simulink model "ElectroHydraulicActuator"  (R2024b)
settings: Solver=VariableStepAuto  StartTime=0.0  StopTime=25  RelTol=1e-3
undefined symbols (not defined in the file or in its folder): B, J, Ke, Kt, L, R
libraries: SignalEditorBlockLib x1
settings Model: Creator=eshwa  LastModifiedBy=eshwa

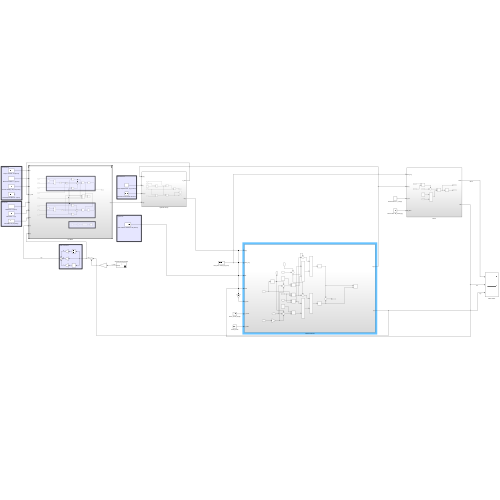
[thumbnail: Simulink's stored preview of the top-level diagram]
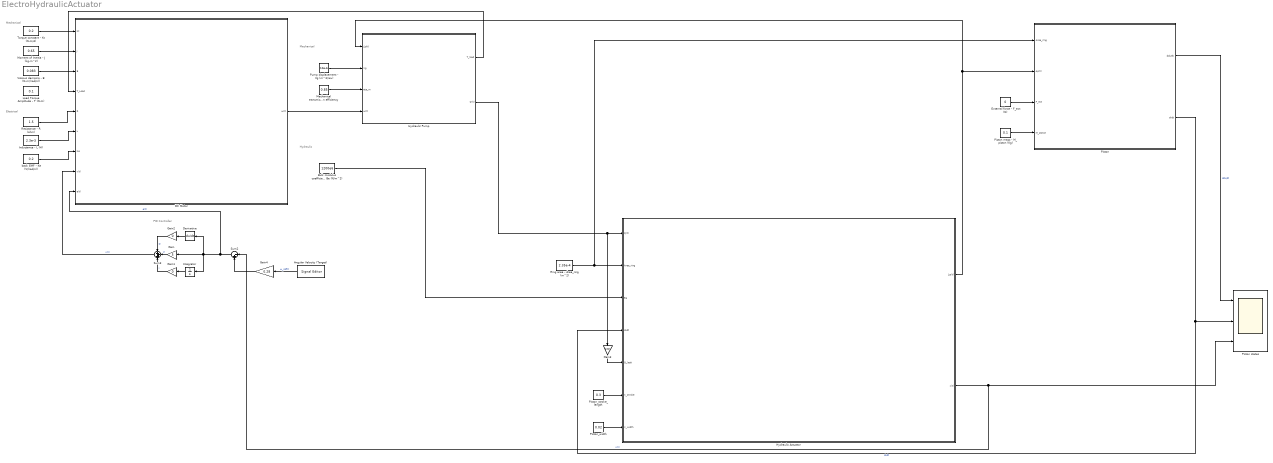
== system ElectroHydraulicActuator ==
  note: Mechanical
  note: PID Controller
  note: Mechanical
  note: Electrical
  note: Hydraulic
  Angular Velocity (Target) : SignalEditorBlockLib/Signal Editor  FileName=omega_ref.mat  ActiveScenario=Scenario  ActiveSignal=Ramp  IsBus=off  OutputBusObjectStr=Bus: BusObject  SampleTime=0  Interpolate=off  ZeroCross=off  OutputAfterFinalValue=Setting to zero  Unit=inherit  PreserveSignalName=on  ApplySigPropsToAllScenarios=on  ApplySigPropsToAllSignals=off
  Bulk modulus coefficient - Be (N/m^2) : Constant  Value=1200e6
  DC Motor : Subsystem
  Derivative : Derivative
  External force - F_ext (N) : Constant  Value=0
  Gain : Gain  Gain=5
  Gain1 : Gain  Gain=0
  Gain2 : Gain  Gain=0
  Gain3 : Gain  Gain=0.02
  Gain4 : Gain  Gain=0.28
  Hydraulic Actuator : Subsystem
  Hydraulic Pump : Subsystem
  Inductance - L (H) : Constant  Value=2.3e-3
  Integrator : Integrator
  Load Torque Amplitude - T (N-m) : Constant  Value=0.1
  Mechanical transmission efficiency : Constant  Value=0.85
  Moment of Inertia - J (kg-m^2) : Constant  Value=0.65
  Piston : Subsystem
  Piston mass - M_piston (Kg) : Constant  Value=0.1
  Piston states : Scope  NumInputPorts=3
  Piston_stroke_length : Constant  Value=0.3
  Piston_width : Constant  Value=0.02
  Pump displacement - Vg (m^3/rev) : Constant  Value=10e-6
  Resistance - R (ohm) : Constant  Value=1.5
  Ring area - Area_ring (m^2) : Constant  Value=2.35e-4
  Sum2 : Sum  Inputs=|-+
  Sum3 : Sum  Inputs=+++
  Torque constant - Kt (N-m/A) : Constant  Value=0.2
  Viscous damping - B (N-m/(rad/s)) : Constant  Value=0.083
  back EMF - Ke (V/(rad/s)) : Constant  Value=0.2
  wires:
  Integrator/1 -> Gain1/1
  Derivative/1 -> Gain2/1
  Gain1/1 -> Sum3/3  "I"
  Gain/1 -> Sum3/2  "P"
  Gain2/1 -> Sum3/1  "D"
  Torque constant - Kt (N-m/A)/1 -> DC Motor/1(Kt)
  Moment of Inertia - J (kg-m^2)/1 -> DC Motor/2(J)
  Viscous damping - B (N-m/(rad/s))/1 -> DC Motor/3(B)
  Resistance - R (ohm)/1 -> DC Motor/5(R)
  Inductance - L (H)/1 -> DC Motor/6(L)
  Sum3/1 -> DC Motor/8(v(t))  "v(t)"
  back EMF - Ke (V/(rad/s))/1 -> DC Motor/7(Ke)
  DC Motor/1(ω(t)) -> Hydraulic Pump/4(ω(t))
  Sum2/1 -> Integrator/1, Derivative/1, Gain/1, DC Motor/9(e(t))  "e(t)"
  Angular Velocity (Target)/1 -> Gain4/1  "ω_ref(t)"
  Pump displacement - Vg (m^3/rev)/1 -> Hydraulic Pump/2(Vg)
  Mechanical transmission efficiency/1 -> Hydraulic Pump/3(eta_m)
  Hydraulic Pump/1(T_load) -> DC Motor/4(T_Load)
  Ring area - Area_ring (m^2)/1 -> Hydraulic Actuator/2(Area_ring), Piston/1(Area_ring)
  Hydraulic Pump/2(Q(t)) -> Gain3/1, Hydraulic Actuator/1(Q(t))
  Bulk modulus coefficient - Be (N/m^2)/1 -> Hydraulic Actuator/3(Ba)
  Piston_stroke_length/1 -> Hydraulic Actuator/6(X_stroke)
  Piston_width/1 -> Hydraulic Actuator/7(X_width)
  Hydraulic Actuator/1(∆p(t)) -> Piston/2(∆p(t)), Hydraulic Pump/1(∆p(t))
  External force - F_ext (N)/1 -> Piston/3(F_ext)
  Piston mass - M_piston (Kg)/1 -> Piston/4(M_piston)
  Piston/2(dxdt) -> Piston states/2, Hydraulic Actuator/4(dxdt)  "dxdt"
  Gain3/1 -> Hydraulic Actuator/5(Q_leak)
  Hydraulic Actuator/2(x(t)) -> Sum2/1, Piston states/3  "x(t)"
  Piston/1(ddx/dt) -> Piston states/1  "ddx/dt"
  Gain4/1 -> Sum2/2

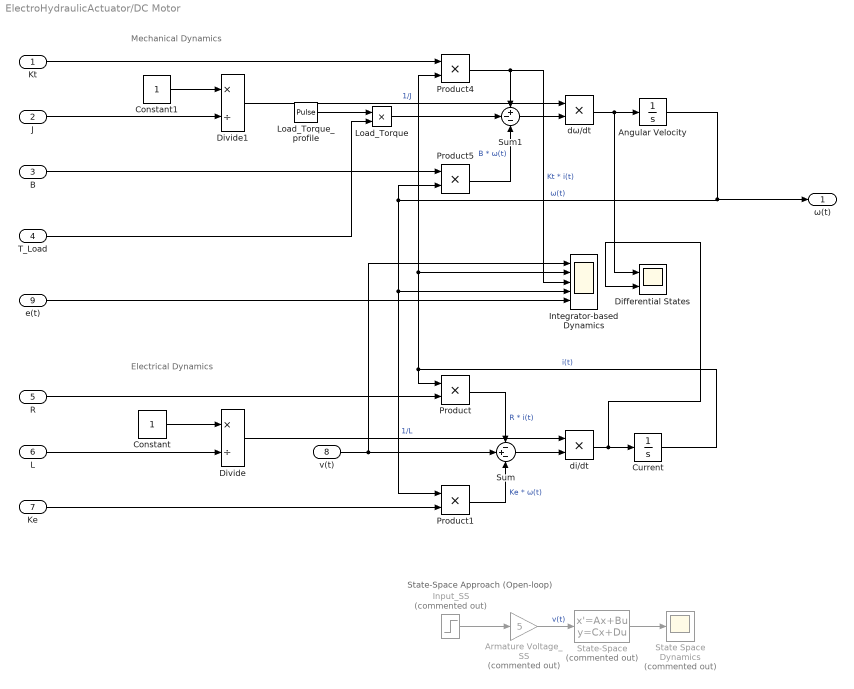
== system ElectroHydraulicActuator/DC Motor ==
  note: Electrical Dynamics
  note: Mechanical Dynamics
  note: State-Space Approach (Open-loop)
  Kt : Inport
  J : Inport  Port=2
  B : Inport  Port=3
  T_Load : Inport  Port=4
  R : Inport  Port=5
  L : Inport  Port=6
  Ke : Inport  Port=7
  v(t) : Inport  Port=8
  e(t) : Inport  Port=9
  Angular Velocity : Integrator
  Armature Voltage_SS : Gain  Commented=on  Gain=5
  Constant : Constant
  Constant1 : Constant
  Current : Integrator
  Differential States : Scope  NumInputPorts=2
  Divide : Product  Inputs=*/
  Divide1 : Product  Inputs=*/
  Input_SS : Step  Commented=on  Time=4  SampleTime=0
  Integrator-based Dynamics : Scope  NumInputPorts=5
  Load_Torque : Product
  Load_Torque_profile : DiscretePulseGenerator  PulseType=Time based  Period=25  PulseWidth=60  PhaseDelay=5
  Product{,1,4..5} (4 alike) : Product
  State Space Dynamics : Scope  Commented=on
  State-Space : StateSpace  Commented=on  A=[-R/L, -Ke/L; Kt/J, -B/J]  B=[1/L; 0]  C=eye(2)  D=[0; 0]  InitialCondition=0  ContinuousStateAttributes={'current', 'velocity'}
  Sum : Sum  Inputs=-+-
  Sum1 : Sum  Inputs=+--
  di/dt : Product
  dω/dt : Product
  ω(t) : Outport
  wires:
  Current/1 -> Product4/2, Integrator-based Dynamics/2, Product/1  "i(t)"
  Product5/1 -> Sum1/3  "B * ω(t)"
  di/dt/1 -> Differential States/2, Current/1
  Load_Torque/1 -> Sum1/2
  Sum1/1 -> dω/dt/2
  dω/dt/1 -> Differential States/1, Angular Velocity/1
  Angular Velocity/1 -> Product1/1, Integrator-based Dynamics/4, Product5/2, ω(t)/1  "ω(t)"
  Product1/1 -> Sum/3  "Ke * ω(t)"
  Product/1 -> Sum/1  "R * i(t)"
  Product4/1 -> Integrator-based Dynamics/3, Sum1/1  "Kt * i(t)"
  Constant1/1 -> Divide1/1
  e(t)/1 -> Integrator-based Dynamics/5
  Constant/1 -> Divide/1
  J/1 -> Divide1/2
  Divide1/1 -> dω/dt/1  "1/J"
  v(t)/1 -> Sum/2, Integrator-based Dynamics/1
  Sum/1 -> di/dt/2
  Divide/1 -> di/dt/1  "1/L"
  Load_Torque_profile/1 -> Load_Torque/1
  Ke/1 -> Product1/2
  L/1 -> Divide/2
  Kt/1 -> Product4/1
  B/1 -> Product5/1
  R/1 -> Product/2
  Armature Voltage_SS/1 -> State-Space/1  "v(t)"
  Input_SS/1 -> Armature Voltage_SS/1
  State-Space/1 -> State Space Dynamics/1
  T_Load/1 -> Load_Torque/2

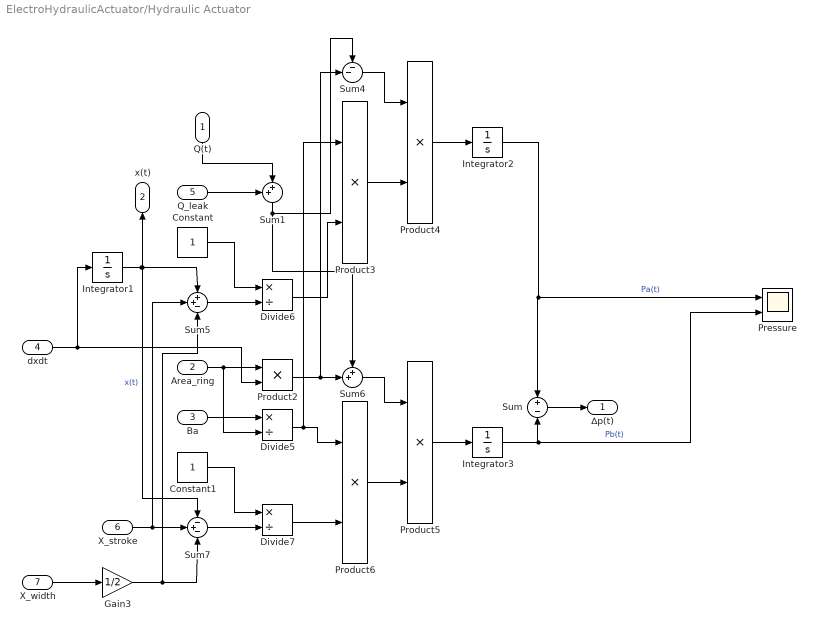
== system ElectroHydraulicActuator/Hydraulic Actuator ==
  Q(t) : Inport
  Area_ring : Inport  Port=2
  Ba : Inport  Port=3
  dxdt : Inport  Port=4
  Q_leak : Inport  Port=5
  X_stroke : Inport  Port=6
  X_width : Inport  Port=7
  Constant : Constant
  Constant1 : Constant
  Divide5 : Product  Inputs=*/
  Divide6 : Product  Inputs=*/
  Divide7 : Product  Inputs=*/
  Gain3 : Gain  Gain=1/2
  Integrator1 : Integrator
  Integrator2 : Integrator  InitialCondition=12.5e6
  Integrator3 : Integrator  InitialCondition=12.5e6
  Pressure : Scope  NumInputPorts=2
  Product{2..6} (5 alike) : Product
  Sum : Sum  Inputs=+-
  Sum1 : Sum  Inputs=++|
  Sum4 : Sum  Inputs=--|
  Sum5 : Sum  Inputs=++-
  Sum6 : Sum  Inputs=++|
  Sum7 : Sum  Inputs=-+-
  ∆p(t) : Outport
  x(t) : Outport  Port=2
  wires:
  Q(t)/1 -> Sum1/2
  dxdt/1 -> Product2/2, Integrator1/1
  Sum/1 -> ∆p(t)/1
  Q_leak/1 -> Sum1/1
  X_stroke/1 -> Sum5/2, Sum7/2
  X_width/1 -> Gain3/1
  Integrator1/1 -> Sum7/1, Sum5/1, x(t)/1  "x(t)"
  Sum6/1 -> Product5/1
  Gain3/1 -> Sum7/3, Sum5/3
  Constant/1 -> Divide6/1
  Divide6/1 -> Product3/2
  Sum5/1 -> Divide6/2
  Area_ring/1 -> Product2/1, Divide5/2
  Ba/1 -> Divide5/1
  Constant1/1 -> Divide7/1
  Divide7/1 -> Product6/2
  Sum7/1 -> Divide7/2
  Sum1/1 -> Sum6/1, Sum4/1
  Product2/1 -> Sum4/2, Sum6/2
  Divide5/1 -> Product6/1, Product3/1
  Sum4/1 -> Product4/1
  Product3/1 -> Product4/2
  Product6/1 -> Product5/2
  Product4/1 -> Integrator2/1
  Product5/1 -> Integrator3/1
  Integrator2/1 -> Sum/1, Pressure/1  "Pa(t)"
  Integrator3/1 -> Pressure/2, Sum/2  "Pb(t)"

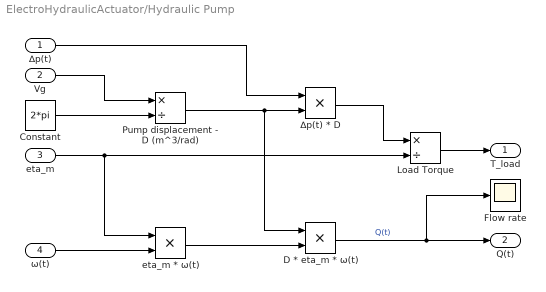
== system ElectroHydraulicActuator/Hydraulic Pump ==
  ∆p(t) : Inport
  Vg : Inport  Port=2
  eta_m : Inport  Port=3
  ω(t) : Inport  Port=4
  Constant : Constant  Value=2*pi
  D * eta_m * ω(t) : Product
  Flow rate : Scope
  Load Torque : Product  Inputs=*/
  Pump displacement - D (m^3/rad) : Product  Inputs=*/
  eta_m * ω(t) : Product
  ∆p(t) * D : Product
  T_load : Outport
  Q(t) : Outport  Port=2
  wires:
  ∆p(t) * D/1 -> Load Torque/1
  Vg/1 -> Pump displacement - D (m^3/rad)/1
  Constant/1 -> Pump displacement - D (m^3/rad)/2
  eta_m/1 -> Load Torque/2, eta_m * ω(t)/1
  eta_m * ω(t)/1 -> D * eta_m * ω(t)/2
  ∆p(t)/1 -> ∆p(t) * D/1
  Pump displacement - D (m^3/rad)/1 -> D * eta_m * ω(t)/1, ∆p(t) * D/2
  ω(t)/1 -> eta_m * ω(t)/2
  D * eta_m * ω(t)/1 -> Flow rate/1, Q(t)/1  "Q(t)"
  Load Torque/1 -> T_load/1

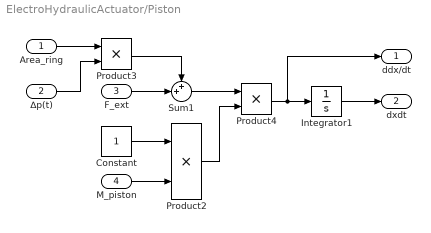
== system ElectroHydraulicActuator/Piston ==
  Area_ring : Inport
  ∆p(t) : Inport  Port=2
  F_ext : Inport  Port=3
  M_piston : Inport  Port=4
  Constant : Constant
  Integrator1 : Integrator
  Product2 : Product
  Product3 : Product
  Product4 : Product
  Sum1 : Sum  Inputs=++|
  ddx/dt : Outport
  dxdt : Outport  Port=2
  wires:
  Product2/1 -> Product4/2
  Sum1/1 -> Product4/1
  Area_ring/1 -> Product3/1
  Constant/1 -> Product2/1
  F_ext/1 -> Sum1/2
  Product3/1 -> Sum1/1
  ∆p(t)/1 -> Product3/2
  M_piston/1 -> Product2/2
  Product4/1 -> ddx/dt/1, Integrator1/1
  Integrator1/1 -> dxdt/1
